simulink model "controlador_LPV_v2"  (R2018b)
settings: Solver=FixedStepAuto  StartTime=0.0  StopTime=7000  FixedStep=T  RelTol=1e-3
values from neighbouring files (symbols this model uses):
  rho = 25    [dim_step.m]
  s_step = 0.02    [dim_step.m]
  T = 5.2632    [dim_step.m]
undefined symbols (not defined in the file or in its folder): K1_, K2_, Ka_, sp
libraries: simulink x1
settings Model: Creator=tarsis  LastModifiedBy=tarsis
settings DebuggingCC: UnderSpecifiedDimensionMsg=warning

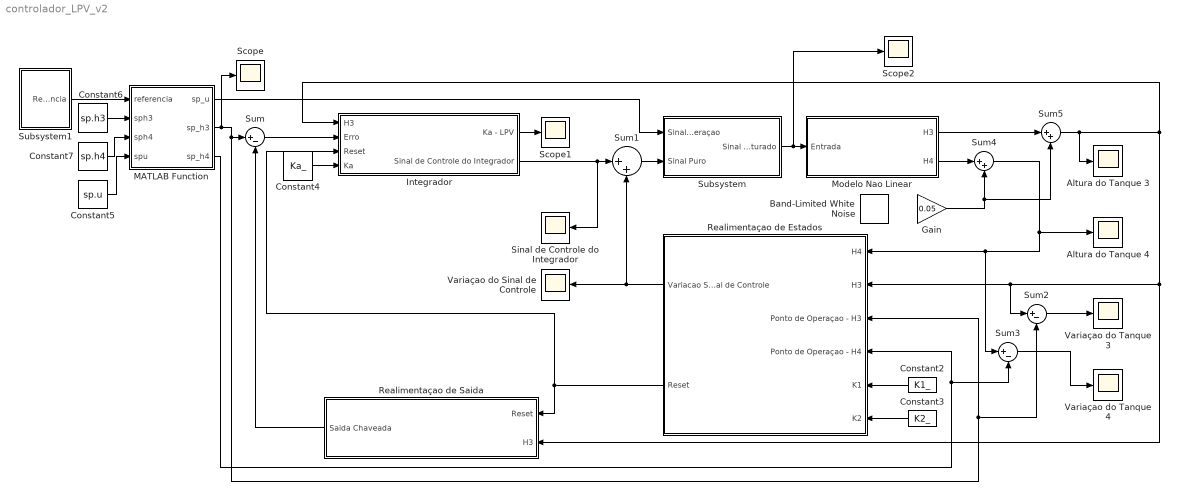
== system controlador_LPV_v2 ==
  Altura do Tanque 3 : Scope
  Altura do Tanque 4 : Scope
  Band-Limited White Noise : simulink/Sources/Band-Limited White Noise  Cov=[0.1]  Ts=3*T  seed=[23341]
  Constant2 : Constant  Value=K1_  VectorParams1D=off
  Constant3 : Constant  Value=K2_  VectorParams1D=off
  Constant4 : Constant  Value=Ka_  VectorParams1D=off
  Constant5 : Constant  Value=sp.u  VectorParams1D=off
  Constant6 : Constant  Value=sp.h3  VectorParams1D=off
  Constant7 : Constant  Value=sp.h4  VectorParams1D=off
  Gain : Gain  Gain=0.05
  Integrador : Subsystem
  MATLAB Function : MATLAB Function  TreatAsAtomicUnit=on
  Modelo Nao Linear : Subsystem
  Realimentaçao de Estados : Subsystem
  Realimentaçao de Saida : Subsystem
  Scope : Scope
  Scope1 : Scope
  Scope2 : Scope
  Sinal de Controle do Integrador : Scope
  Subsystem : Subsystem
  Subsystem1 : Subsystem
  Sum : Sum  Inputs=|+-
  Sum1 : Sum  Inputs=|++
  Sum2 : Sum  Inputs=|+-
  Sum3 : Sum  Inputs=|+-
  Sum4 : Sum  Inputs=|++
  Sum5 : Sum  Inputs=|++
  Variaçao do Sinal de Controle : Scope
  Variaçao do Tanque 3 : Scope
  Variaçao do Tanque 4 : Scope
  wires:
  Realimentaçao de Saida/1(Saida Chaveada) -> Sum/2
  Sum/1 -> Integrador/2(Erro)
  Realimentaçao de Estados/1(Variacao Sinal de Controle) -> Sum1/2, Variaçao do Sinal de Controle/1
  Integrador/2(Sinal de Controle do Integrador) -> Sum1/1, Sinal de Controle do Integrador/1
  Realimentaçao de Estados/2(Reset) -> Integrador/3(Reset), Realimentaçao de Saida/1(Reset)
  Sum1/1 -> Subsystem/2(Sinal Puro)
  Subsystem/1(Sinal Saturado) -> Scope2/1, Modelo Nao Linear/1(Entrada)
  Constant2/1 -> Realimentaçao de Estados/5(K1)
  Constant3/1 -> Realimentaçao de Estados/6(K2)
  Constant4/1 -> Integrador/4(Ka)
  Modelo Nao Linear/1(H3) -> Sum5/1
  Sum2/1 -> Variaçao do Tanque 3/1
  Sum3/1 -> Variaçao do Tanque 4/1
  Subsystem1/1(Referencia) -> MATLAB Function/1(referencia)
  Constant6/1 -> MATLAB Function/2(sph3)
  Constant7/1 -> MATLAB Function/3(sph4)
  Constant5/1 -> MATLAB Function/4(spu)
  MATLAB Function/1(sp_u) -> Subsystem/1(Sinal de Operaçao)
  MATLAB Function/3(sp_h4) -> Sum3/2, Realimentaçao de Estados/4(Ponto de Operaçao - H4)
  MATLAB Function/2(sp_h3) -> Scope/1, Sum/1, Sum2/2, Realimentaçao de Estados/3(Ponto de Operaçao - H3)
  Modelo Nao Linear/2(H4) -> Sum4/1
  Sum4/1 -> Sum3/1, Realimentaçao de Estados/1(H4), Altura do Tanque 4/1
  Sum5/1 -> Integrador/1(H3), Realimentaçao de Saida/2(H3), Sum2/1, Realimentaçao de Estados/2(H3), Altura do Tanque 3/1
  Gain/1 -> Sum5/2, Sum4/2
  Integrador/1(Ka - LPV) -> Scope1/1

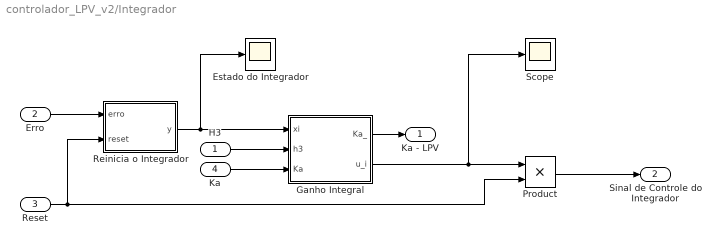
== system controlador_LPV_v2/Integrador ==
  H3 : Inport
  Erro : Inport  Port=2
  Reset : Inport  Port=3
  Ka : Inport  Port=4
  Estado do Integrador : Scope
  Ganho Integral : MATLAB Function  TreatAsAtomicUnit=on
  Product : Product
  Reinicia o Integrador : MATLAB Function  TreatAsAtomicUnit=on  SystemSampleTime=T
  Scope : Scope
  Ka - LPV : Outport
  Sinal de Controle do Integrador : Outport  Port=2
  wires:
  H3/1 -> Ganho Integral/2(h3)
  Reinicia o Integrador/1(y) -> Estado do Integrador/1, Ganho Integral/1(xi)
  Reset/1 -> Reinicia o Integrador/2(reset), Product/2
  Ganho Integral/2(u_i) -> Scope/1, Product/1
  Product/1 -> Sinal de Controle do Integrador/1
  Erro/1 -> Reinicia o Integrador/1(erro)
  Ka/1 -> Ganho Integral/3(Ka)
  Ganho Integral/1(Ka_) -> Ka - LPV/1

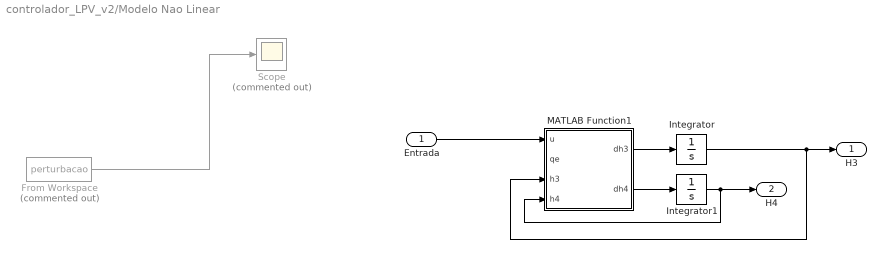
== system controlador_LPV_v2/Modelo Nao Linear ==
  Entrada : Inport
  From Workspace : FromWorkspace  Commented=on  VariableName=perturbacao  SampleTime=T  Interpolate=off  OutputAfterFinalValue=Setting to zero
  Integrator : Integrator
  Integrator1 : Integrator
  MATLAB Function1 : MATLAB Function  TreatAsAtomicUnit=on
  Scope : Scope  Commented=on
  H3 : Outport
  H4 : Outport  Port=2
  wires:
  Integrator1/1 -> H4/1, MATLAB Function1/4(h4)
  Entrada/1 -> MATLAB Function1/1(u)
  MATLAB Function1/2(dh4) -> Integrator1/1
  Integrator/1 -> H3/1, MATLAB Function1/3(h3)
  MATLAB Function1/1(dh3) -> Integrator/1
  From Workspace/1 -> Scope/1

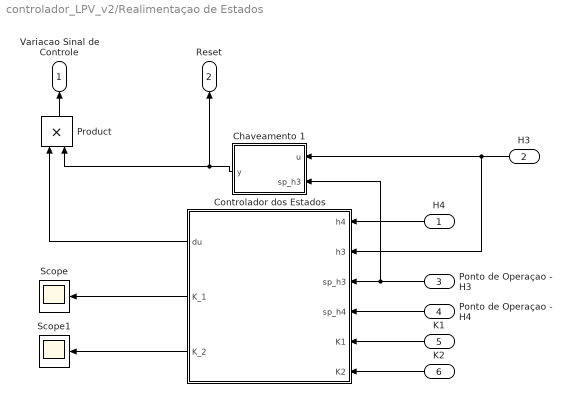
== system controlador_LPV_v2/Realimentaçao de Estados ==
  H4 : Inport
  H3 : Inport  Port=2
  Ponto de Operaçao - H3 : Inport  Port=3
  Ponto de Operaçao - H4 : Inport  Port=4
  K1 : Inport  Port=5
  K2 : Inport  Port=6
  Chaveamento 1 : MATLAB Function  TreatAsAtomicUnit=on
  Controlador dos Estados : MATLAB Function  TreatAsAtomicUnit=on  SystemSampleTime=T
  Product : Product
  Scope : Scope
  Scope1 : Scope
  Variacao Sinal de Controle : Outport
  Reset : Outport  Port=2
  wires:
  Chaveamento 1/1(y) -> Reset/1, Product/2
  H4/1 -> Controlador dos Estados/1(h4)
  H3/1 -> Controlador dos Estados/2(h3), Chaveamento 1/1(u)
  Product/1 -> Variacao Sinal de Controle/1
  Controlador dos Estados/1(du) -> Product/1
  Ponto de Operaçao - H3/1 -> Chaveamento 1/2(sp_h3), Controlador dos Estados/3(sp_h3)
  Ponto de Operaçao - H4/1 -> Controlador dos Estados/4(sp_h4)
  K1/1 -> Controlador dos Estados/5(K1)
  K2/1 -> Controlador dos Estados/6(K2)
  Controlador dos Estados/2(K_1) -> Scope/1
  Controlador dos Estados/3(K_2) -> Scope1/1

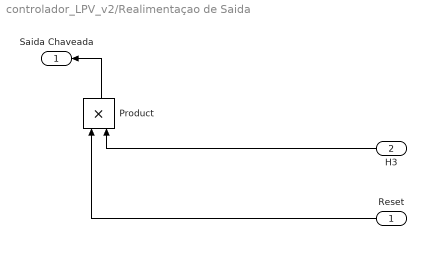
== system controlador_LPV_v2/Realimentaçao de Saida ==
  Reset : Inport
  H3 : Inport  Port=2
  Product : Product
  Saida Chaveada : Outport
  wires:
  H3/1 -> Product/2
  Product/1 -> Saida Chaveada/1
  Reset/1 -> Product/1

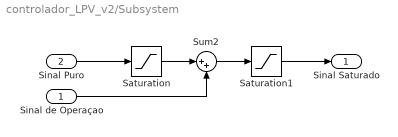
== system controlador_LPV_v2/Subsystem ==
  Sinal de Operaçao : Inport
  Sinal Puro : Inport  Port=2
  Saturation : Saturate  UpperLimit=rho  LowerLimit=-rho
  Saturation1 : Saturate  UpperLimit=2*rho  LowerLimit=0
  Sum2 : Sum  Inputs=|++
  Sinal Saturado : Outport
  wires:
  Saturation/1 -> Sum2/1
  Sinal de Operaçao/1 -> Sum2/2
  Sum2/1 -> Saturation1/1
  Sinal Puro/1 -> Saturation/1
  Saturation1/1 -> Sinal Saturado/1

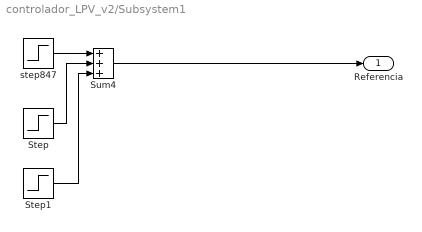
== system controlador_LPV_v2/Subsystem1 ==
  Step : Step  Time=3500  After=s_step  SampleTime=0
  Step1 : Step  Time=5000  After=s_step  SampleTime=0
  Sum4 : Sum  Inputs=|+|+|+|
  step847 : Step  Time=0  After=sp.h3(1)  SampleTime=0
  Referencia : Outport
  wires:
  Step1/1 -> Sum4/3
  step847/1 -> Sum4/1
  Step/1 -> Sum4/2
  Sum4/1 -> Referencia/1

== matlab function controlador_LPV_v2/Modelo Nao Linear/MATLAB Function1 ==
  data: u input; qe input; dh3 output; h3 input; h4 input; dh4 output
function [dh3,dh4] = fcn(u,qe,h3,h4)
qi = (16.4*u + 357.3)*1e-6;
q12 = 33.51e-4*(h4 - h3) + 43.12e-5;
qout = (87.07e-5*sqrt(h3) + 30.99e-5);
A1 = (pi*(31)^2)*1e-4;
A2 = - 0.88629272879272778105782609278436*h3^16 + 6.0267905557905489111932174309337*h3^15 - 20.80464391736738395516887057851*h3^14 + 47.68494439008527766774004035511*h3^13 - 82.573907447205791291786792565001*h3^12 + 116.28257881925208875326233578017*h3^11 - 139.30893428077013388311346843447*h3^10 + 144.80767028205944702410747888441*h3^9 - 129.2475129476872169884635810807*h3^8 + 96.099152680911332924853135955618*h3^7 - 55.593870964701796673125553833866*h3^6 + 21.451550218200266654046211819752*h3^5 - 5.9275208717979510465216954484015*h3^4 + 3.9856416105248966168880953176109*h3^3 - 2.0902185091906828919771687989635*h3^2 - 0.061481774188906647716430580264178*h3 + 0.32722421068834535751546101783638;
dh4 = (qi - q12)/A1;
dh3 = (q12 - qout + qe)/A2;

== matlab function controlador_LPV_v2/Integrador/Ganho Integral ==
  data: Ka_ output; xi input; u_i output; h3 input; Ka input
function [Ka_,u_i] = fcn(xi,h3,Ka)

Ka_ = h3*0.05*(Ka(2) - Ka(1)) + 2.4*Ka(1) - 1.4*Ka(2);
u_i = xi*Ka_;

== matlab function controlador_LPV_v2/Realimentaçao de Estados/Controlador dos Estados ==
  data: h4 input; h3 input; du output; sp_h3 input; sp_h4 input; K1 input; K2 input; K_1 output; K_2 output
function [du,K_1,K_2]  = fcn(h4,h3,sp_h3,sp_h4,K1,K2)
% Saída do Modelo não Linear
h = [h4 h3]';
% Pontos de Operação
sp_h = [sp_h4 sp_h3]';
% Equação do Ganho LPV em função de alfa
K = h3*0.05*(K2 - K1) + 2.4*K1 - 1.4*K2;
% Separando os valores de K
K_1 = K(1);
K_2 = K(2);
% Realimentação do Estados
du = K*(h - sp_h);

== matlab function controlador_LPV_v2/Realimentaçao de Estados/Chaveamento 1 ==
  settings: updateMethod=DISCRETE
  data: u input; y output; sp_h3 input
function y = fcn(u,sp_h3)
persistent d
if isempty(d)
    d = true;
end

if u<0.95*sp_h3 && d==true
    y = 0;
else
    d = false;
    y = 1;
end

== matlab function controlador_LPV_v2/MATLAB Function ==
  data: sp_u output; referencia input; sph3 input; sph4 input; spu input; sp_h3 output; sp_h4 output
function [sp_u,sp_h3,sp_h4]  = fcn(referencia,sph3,sph4,spu)
if referencia == sph3(1)
    sp_u = spu(1);
    sp_h3 = sph3(1);
    sp_h4 = sph4(1);
elseif referencia > sph3(1) && referencia < sph3(3)
    sp_u = spu(1);
    sp_h3 = sph3(2);
    sp_h4 = sph4(2);
else
    sp_u = spu(1);
    sp_h3 = sph3(3);
    sp_h4 = sph4(3);
end

== matlab function controlador_LPV_v2/Integrador/Reinicia o Integrador ==
  settings: updateMethod=DISCRETE
  data: erro input; y output; reset input
function y = fcn(erro,reset)
% Estado do integrador
persistent xi
% Variável do Reset
persistent d
% Criando variáveis persistentes
if isempty(d)
    d = true;
end
if isempty(xi)
    xi = 0;
end
% Reset do integrador
if reset == 1 && d == true
    d = false;
    xi = 0;
end
% Ação integral
xi = erro + xi;
y = xi;
